simulink model "Part2_4QAM"  (R2017a)
settings: Solver=VariableStepAuto  StartTime=0.0  StopTime=1  RelTol=1e-3
libraries: commutil2 x1, commrandsrc3 x1
settings Model: Creator=Marine  LastModifiedBy=mhuynh7
settings SFSimCC: SimUseLocalCustomCode=on
settings RTWCC: RTWUseLocalCustomCode=on

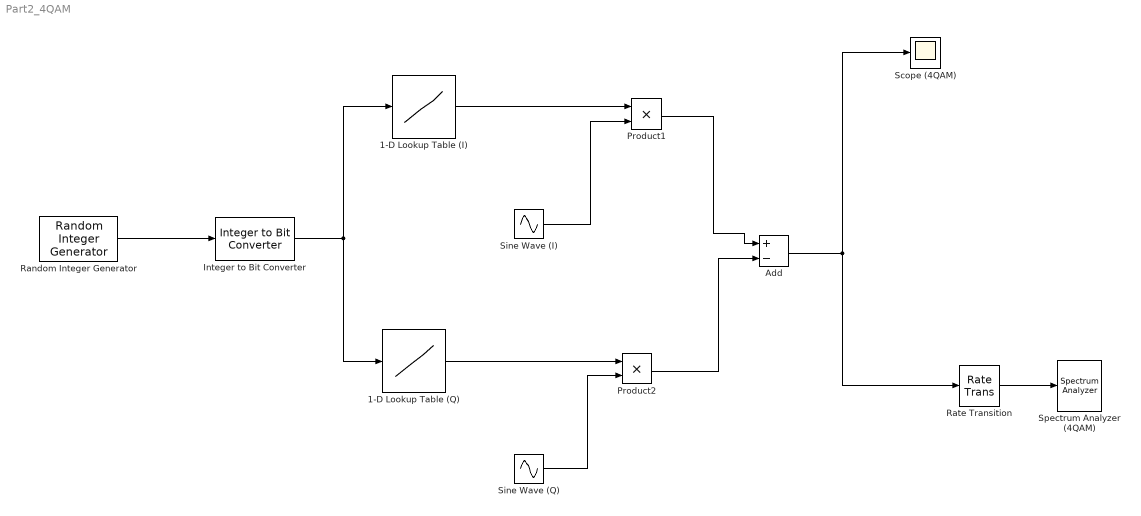
== system Part2_4QAM ==
  1-D Lookup Table (I) : Lookup_n-D  NumberOfTableDimensions=1  BreakpointsForDimension1=[0,1]  Table=[-sqrt(0.5),sqrt(0.5)]  InternalRulePriority=Speed  RndMeth=Simplest  InputSameDT=on
  1-D Lookup Table (Q) : Lookup_n-D  NumberOfTableDimensions=1  BreakpointsForDimension1=[0,1]  Table=[-sqrt(0.5), sqrt(0.5)]  InternalRulePriority=Speed  RndMeth=Simplest  InputSameDT=on
  Add : Sum  Inputs=+-
  Integer to Bit Converter : commutil2/Integer to Bit Converter  nbits=3  signedInputValues=Unsigned  bitOrder=MSB first  outDtype=Inherit via internal rule
  Product1 : Product
  Product2 : Product
  Random Integer Generator : commrandsrc3/Random Integer Generator  SetSize=8  SeedSource=Auto  Seed=0  SampleTime=1  SamplesPerFrame=1  OutputDataType=double  SimulateUsing=Interpreted execution
  Rate Transition : RateTransition  OutPortSampleTime=0.5e-4
  Scope (4QAM) : Scope
  Sine Wave (I) : Sin  SineType=Sample based  Samples=5000  SampleTime=1e-7  Offset=1250
  Sine Wave (Q) : Sin  SineType=Sample based  Samples=5000  SampleTime=1e-7
  Spectrum Analyzer (4QAM) : SpectrumAnalyzer
  wires:
  Rate Transition/1 -> Spectrum Analyzer (4QAM)/1
  Sine Wave (I)/1 -> Product1/2
  1-D Lookup Table (I)/1 -> Product1/1
  Product1/1 -> Add/1
  Sine Wave (Q)/1 -> Product2/2
  1-D Lookup Table (Q)/1 -> Product2/1
  Product2/1 -> Add/2
  Add/1 -> Rate Transition/1, Scope (4QAM)/1
  Random Integer Generator/1 -> Integer to Bit Converter/1
  Integer to Bit Converter/1 -> 1-D Lookup Table (Q)/1, 1-D Lookup Table (I)/1
